simulink model "GFL_mask"  (R2024b)
settings: Solver=ode3  StartTime=0.0  StopTime=20  FixedStep=1e-5  RelTol=1e-3  EnableMultiTasking=on
InitFcn:
  | Ts=5e-6;
values from neighbouring files (symbols this model uses):
  c_f = 0.06    [GFL_compare.m]    (also in dqscan.m; fun00_GFL_pu_2_normial.m = c_f*Cb; fun01_GFL_Small_Signal.m = c_f*Cb)
  fb = 60    [GFL_compare.m]    (also in dqscan.m)
  fpt = fp1    [dqscan.m]
  ki_i = ki_i_pu*Vb_p_ph/Ib_p_ph    [fun00_GFL_pu_2_normial.m]    (also in fun01_GFL_Small_Signal.m)
  ki_p = ki_p_pu/Sb*Ib_p_ph    [fun00_GFL_pu_2_normial.m]    (also in fun01_GFL_Small_Signal.m)
  ki_pll = 377.7    [GFL_compare.m]    (also in dqscan.m; fun00_GFL_pu_2_normial.m = ki_pll/Vb_p_ph; fun01_GFL_Small_Signal.m = ki_pll/Vb_p_ph)
  ki_q = ki_q_pu/Sb*Ib_p_ph    [fun00_GFL_pu_2_normial.m]    (also in fun01_GFL_Small_Signal.m)
  kp_i = kp_i_pu*Vb_p_ph/Ib_p_ph    [fun00_GFL_pu_2_normial.m]    (also in fun01_GFL_Small_Signal.m)
  kp_p = kp_p_pu/Sb*Ib_p_ph    [fun00_GFL_pu_2_normial.m]    (also in fun01_GFL_Small_Signal.m)
  kp_pll = 27.5    [GFL_compare.m]    (also in dqscan.m; fun00_GFL_pu_2_normial.m = kp_pll/Vb_p_ph; fun01_GFL_Small_Signal.m = kp_pll/Vb_p_ph)
  kp_q = kp_q_pu/Sb*Ib_p_ph    [fun00_GFL_pu_2_normial.m]    (also in fun01_GFL_Small_Signal.m)
  l_f = 0.05    [GFL_compare.m]    (also in dqscan.m; fun00_GFL_pu_2_normial.m = l_f*Lb; fun01_GFL_Small_Signal.m = l_f*Lb)
  pset = p_set_pu*Sb    [fun00_GFL_pu_2_normial.m]    (also in fun01_GFL_Small_Signal.m)
  qset = q_set_pu*Sb    [fun00_GFL_pu_2_normial.m]    (also in fun01_GFL_Small_Signal.m)
  r_f = 0.01    [GFL_compare.m]    (also in dqscan.m; fun00_GFL_pu_2_normial.m = r_f*Zb; fun01_GFL_Small_Signal.m = r_f*Zb)
  Sb = 50*10^3    (= 50000)    [GFL_compare.m]    (also in dqscan.m)
  Upd = 0    [dqscan.m]
  Upq = 10    [dqscan.m]
  Vb = 690    [GFL_compare.m]    (also in dqscan.m)
  Vdc = 3*Vb_p_ph    [fun00_GFL_pu_2_normial.m]
  w_b = fb*2*pi    (= 376.991118431)    [GFL_compare.m]    (also in dqscan.m; fun00_GFL_pu_2_normial.m = fb*2*pi; fun01_GFL_Small_Signal.m = fb*2*pi)
undefined symbols (not defined in the file or in its folder): DiscIntNeverNeededParam
libraries: spsabctodq0Lib x10, spsThreePhaseVIMeasurementLib x6, slpidlib x5, spsControlledVoltageSourceLib x3, spsThreePhaseSeriesRLCBranchLib x3, spsGroundLib x2, spsdq0toabcLib x2, spsPowerPositiveSequenceLib x1, spsUniversalBridgeLib x1, spsDCVoltageSourceLib x1, spsPLL3phLib x1, spsThreePhaseProgrammableVoltageSourceLib x1
settings Model: SimulationMode=accelerator  Creator=GeZicheng  LastModifiedBy=PEESE_hmqrtt2
settings DataIOCC: SaveFinalState=on  SaveFormat=StructureWithTime  SaveOutput=off  SignalLogging=off  SaveTime=off  ReturnWorkspaceOutputs=off

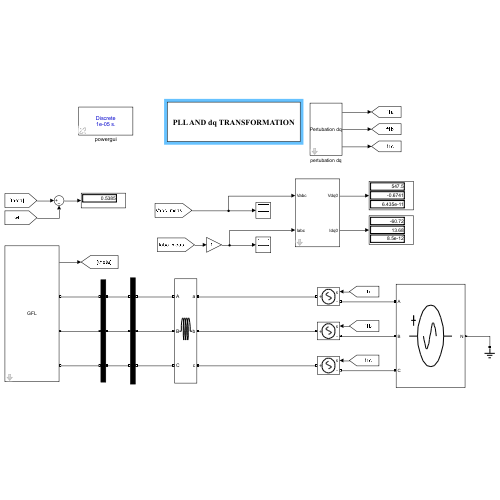
[thumbnail: Simulink's stored preview of the top-level diagram]
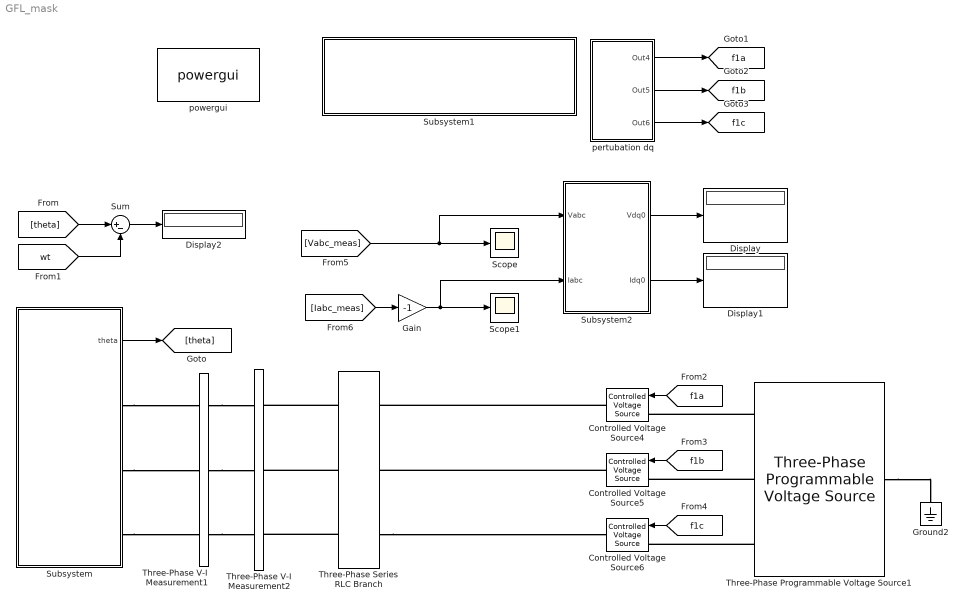
== system GFL_mask ==
  Controlled Voltage Source4 : spsControlledVoltageSourceLib/Controlled Voltage Source  Initialize=on  Source_Type=AC  Amplitude=0  Phase=0  Frequency=0  Measurements=None
  Controlled Voltage Source5 : spsControlledVoltageSourceLib/Controlled Voltage Source  Initialize=on  Source_Type=AC  Amplitude=0  Phase=0  Frequency=0  Measurements=None
  Controlled Voltage Source6 : spsControlledVoltageSourceLib/Controlled Voltage Source  Initialize=on  Source_Type=AC  Amplitude=0  Phase=0  Frequency=0  Measurements=None
  Display : Display
  Display1 : Display
  Display2 : Display
  Gain : Gain  Gain=-1
  Ground2 : spsGroundLib/Ground  LConnTagsString=a
  Scope : Scope
  Scope1 : Scope
  Subsystem : Subsystem  mask{Pnom=Sb, Vnom=Vb, Fnom=fb, Vdc_nom=Vdc, RLC_Filter=[r_f l_f c_f], Pref=pset, Qref=qset, PLL_p=kp_pll, PLL_i=ki_pll, Voltage_P=kp_q, Voltage_I=ki_q, Current_P=kp_i, Current_I=ki_i, Power_P=kp_p, Power_I=ki_p, kf=0.5}
      mask prompts: Pnom "Rated Power(VA)"; Vnom "Rated L-L RMS Voltage(V)"; Fnom "Rated Frequency(Hz)"; Vdc_nom "DC capacitor voltage(V)"; RLC_Filter "Grid-side coupling impedance(p.u.)"; Pref "Power Setting"; Qref "Voltage Setting"; PLL_p "PL Proportional Gain"; PLL_i "PLL Integral Gain"; Voltage_P "Voltage Proportional Gain"; Voltage_I "Voltage Integral Gain"; Current_P "Current Proportional Gain"; Current_I "Current Integral Gain"; Power_P "Power Proportional Gain"; Power_I "Power Integral Gain"; kf "Feedforward Gain"
      mask init:
      | R_f=RLC_Filter(1);
      | L_f=RLC_Filter(2);
      | C_f=RLC_Filter(3);
      mask Display: disp('GFL')
  Subsystem1 : Subsystem
      mask Display: disp('PLL AND dq TRANSFORMATION')
  Subsystem2 : Subsystem
      mask DialogControl ParameterGroupVar Prompt: 参数
  Sum : Sum  Inputs=|+-
  Three-Phase Programmable Voltage Source1 : spsThreePhaseProgrammableVoltageSourceLib/Three-Phase Programmable Voltage Source  PositiveSequence=[Vb 90 fb]  VariationEntity=None  VariationType=Table of time-amplitude pairs  VariationTypeAlt=Step  VariationStep=0.5  VariationRate=10  VariationMagnitude=0.3  VariationFrequency=2  VariationTiming=[1 2]  VariationPhaseA=off  Amplitudes=[1 0.8 1.2 1.0]  TimeValues=[0 0.1 0.15 0.2]  HarmonicGeneration=off  HarmonicA=[3 0.2 -25 0]  HarmonicB=[2 0.15 35 2]  Timing="[0.05  3]"  BusType=swing  Pref=0  Qref=0  Qmin=-inf  Qmax=inf
  Three-Phase Series RLC Branch : spsThreePhaseSeriesRLCBranchLib/Three-Phase Series RLC Branch  LConnTagsString=A|B|C  RConnTagsString=A|B|C  BranchType=L  Resistance=r_f  Inductance=10*l_f  Capacitance=1e-6  Measurements=None
  Three-Phase V-I Measurement1 : spsThreePhaseVIMeasurementLib/Three-Phase V-I Measurement  VoltageMeasurement=phase-to-ground  SetLabelV=on  LabelV=Vabc_o  Vpu=off  VpuLL=off  CurrentMeasurement=yes  SetLabelI=on  LabelI=Iabc_o  Ipu=off  Pbase=100e6  Vbase=500e3  OutputType=Complex  PhasorSimulation=off  PSBequivalent=0
  Three-Phase V-I Measurement2 : spsThreePhaseVIMeasurementLib/Three-Phase V-I Measurement  VoltageMeasurement=phase-to-ground  SetLabelV=on  LabelV=Vabc_meas  Vpu=off  VpuLL=off  CurrentMeasurement=yes  SetLabelI=on  LabelI=Iabc_meas  Ipu=off  Pbase=100e6  Vbase=500e3  OutputType=Complex  PhasorSimulation=off  PSBequivalent=0
  pertubation dq : Subsystem
      mask DialogControl ParameterGroupVar Prompt: 参数
      mask Display: disp('Pertubation dq')
  powergui : spspowerguiLib/powergui  SimulationMode=Discrete  SampleTime=1e-5  frequency=50  Iterations=50  frequencyindice=0  Pbase=100e6  ErrMax=1e-4  UnitsV=kV  UnitsW=MW  buscounter=0  FunctionMessages=off  echomessages=off  EnableUseOfTLC=off  CurrentSourceSwitches=on  DisableSnubberDevices=off  DisableRonSwitches=off  DisableVfSwitches=off  DisplayEquations=off  AutomaticDiscreteSolvers=off  SolverType=Tustin/Backward Euler (TBE)  Interpol=off  ExternalGateDelay=off  methode=off  Ts=0  x0status=blocks  SPID=off  SwTol=0  HookPort=off  NonlinearTolerance=1e-4  nMaxIteration=100  ContinueOnMaxIteration=off  RestoreLinks=warning  ResistiveCurrentMeasurement=off  Frange=[0:2:500]  Ylog=off  Xlog=on  ShowGrid=off  save=off  variable=ZData  structure=0  ZoomFFT=on  StartTime=0.0  cycles=1  DisplayStyle=1  fundamental=60  FreqAxis=off  MaxFrequency=1000  frequencyindicesteady=1  RmsSteady=1  display=off
  tag scope: f1a=global, f1b=global, f1c=global
  wires:
  [Vabc_meas] -> Subsystem2/1(Vabc), Scope/1
  [f1c] -> Controlled Voltage Source6/1
  [f1b] -> Controlled Voltage Source5/1
  [f1a] -> Controlled Voltage Source4/1
  pertubation dq/3(Out6) -> [f1c]
  pertubation dq/1(Out4) -> [f1a]
  pertubation dq/2(Out5) -> [f1b]
  Subsystem2/1(Vdq0) -> Display/1
  Subsystem2/2(Idq0) -> Display1/1
  Gain/1 -> Subsystem2/2(Iabc), Scope1/1
  [theta] -> Sum/1
  [wt] -> Sum/2
  Sum/1 -> Display2/1
  Subsystem/1(theta) -> [theta]
  [Iabc_meas] -> Gain/1
  connections:
  Three-Phase V-I Measurement1/RConn1 -- Three-Phase V-I Measurement2/LConn1
  Three-Phase V-I Measurement1/RConn2 -- Three-Phase V-I Measurement2/LConn2
  Three-Phase V-I Measurement1/RConn3 -- Three-Phase V-I Measurement2/LConn3
  Three-Phase Programmable Voltage Source1/RConn1 -- Controlled Voltage Source4/LConn1
  Three-Phase Programmable Voltage Source1/RConn2 -- Controlled Voltage Source5/LConn1
  Three-Phase Programmable Voltage Source1/RConn3 -- Controlled Voltage Source6/LConn1
  Three-Phase Programmable Voltage Source1/LConn1 -- Ground2/LConn1
  Subsystem/RConn1 -- Three-Phase V-I Measurement1/LConn1
  Subsystem/RConn2 -- Three-Phase V-I Measurement1/LConn2
  Subsystem/RConn3 -- Three-Phase V-I Measurement1/LConn3
  Three-Phase Series RLC Branch/RConn3 -- Controlled Voltage Source6/RConn1
  Controlled Voltage Source5/RConn1 -- Three-Phase Series RLC Branch/RConn2
  Controlled Voltage Source4/RConn1 -- Three-Phase Series RLC Branch/RConn1
  Three-Phase Series RLC Branch/LConn1 -- Three-Phase V-I Measurement2/RConn1
  Three-Phase Series RLC Branch/LConn2 -- Three-Phase V-I Measurement2/RConn2
  Three-Phase Series RLC Branch/LConn3 -- Three-Phase V-I Measurement2/RConn3

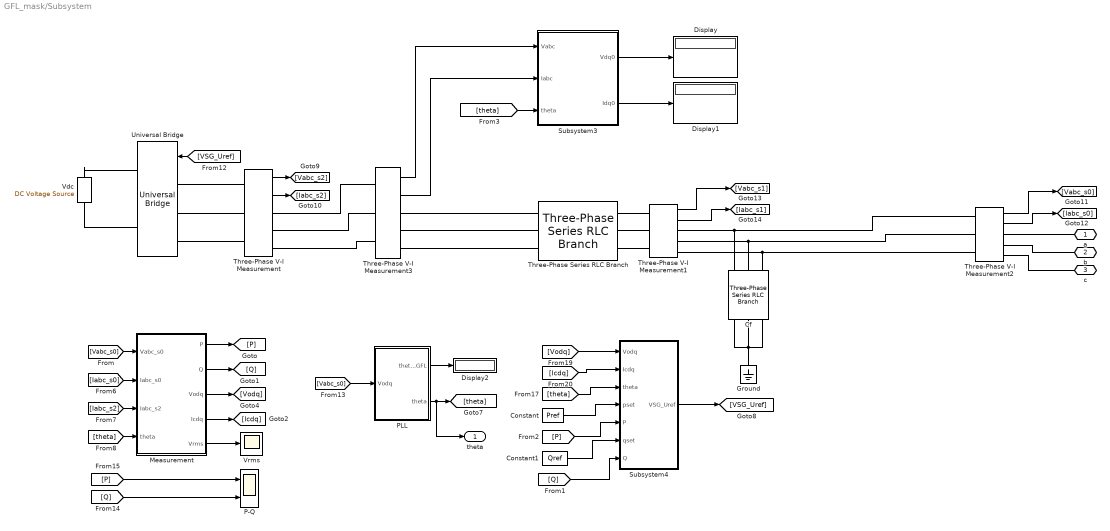
== system GFL_mask/Subsystem ==
  Cf : spsThreePhaseSeriesRLCBranchLib/Three-Phase Series RLC Branch  LConnTagsString=A|B|C  RConnTagsString=A|B|C  BranchType=C  Resistance=0.1  Inductance=1e-3  Capacitance=RLC_Filter(3)  Measurements=None
  Constant : Constant  Value=Pref
  Constant1 : Constant  Value=Qref
  Display : Display
  Display1 : Display
  Display2 : Display
  Ground : spsGroundLib/Ground  LConnTagsString=a
  Measurement : Subsystem
      mask DialogControl ParameterGroupVar Prompt: 参数
  P-Q : Scope  NumInputPorts=2
  PLL : Subsystem
      mask DialogControl ParameterGroupVar Prompt: 参数
  Subsystem3 : Subsystem
      mask DialogControl ParameterGroupVar Prompt: 参数
  Subsystem4 : Subsystem  mask{Voltage_P=Voltage_P, Voltage_I=Voltage_I, Current_P=Current_P, Current_I=Current_I, Power_P=Power_P, Power_I=Power_I, kf=kf}
      mask prompts: Voltage_P "Voltage Proportional Coefficient"; Voltage_I "Voltage Integral Coefficient"; Current_P "Current Proportional Coefficient"; Current_I "Current Integral Coefficient"; Power_P "Power Proportional Coefficient"; Power_I "Power Integral Coefficient"; kf "Feedforward Coeffcient"
      mask DialogControl ParameterGroupVar Prompt: Controller Parameter
  Three-Phase Series RLC Branch : spsThreePhaseSeriesRLCBranchLib/Three-Phase Series RLC Branch  LConnTagsString=A|B|C  RConnTagsString=A|B|C  BranchType=RL  Resistance=RLC_Filter(1)  Inductance=RLC_Filter(2)  Capacitance=1e-6  Measurements=None
  Three-Phase V-I Measurement : spsThreePhaseVIMeasurementLib/Three-Phase V-I Measurement  VoltageMeasurement=phase-to-ground  SetLabelV=off  LabelV=Vabc_s2  Vpu=off  VpuLL=off  CurrentMeasurement=yes  SetLabelI=off  LabelI=Iabc_s2  Ipu=off  Pbase=Pnom  Vbase=Vnom  OutputType=Complex  PhasorSimulation=off  PSBequivalent=0
  Three-Phase V-I Measurement1 : spsThreePhaseVIMeasurementLib/Three-Phase V-I Measurement  VoltageMeasurement=phase-to-ground  SetLabelV=off  LabelV=Vabc_s1  Vpu=off  VpuLL=off  CurrentMeasurement=yes  SetLabelI=off  LabelI=Iabc_s1  Ipu=off  Pbase=Pnom  Vbase=Vnom  OutputType=Complex  PhasorSimulation=off  PSBequivalent=0
  Three-Phase V-I Measurement2 : spsThreePhaseVIMeasurementLib/Three-Phase V-I Measurement  VoltageMeasurement=phase-to-ground  SetLabelV=off  LabelV=Vabc_s0  Vpu=off  VpuLL=off  CurrentMeasurement=yes  SetLabelI=off  LabelI=Iabc_s0  Ipu=off  Pbase=Pnom  Vbase=Vnom  OutputType=Complex  PhasorSimulation=off  PSBequivalent=0
  Three-Phase V-I Measurement3 : spsThreePhaseVIMeasurementLib/Three-Phase V-I Measurement  VoltageMeasurement=phase-to-ground  SetLabelV=off  LabelV=Vabc_s2  Vpu=off  VpuLL=off  CurrentMeasurement=yes  SetLabelI=off  LabelI=Iabc_s2  Ipu=off  Pbase=Pnom  Vbase=Vnom  OutputType=Complex  PhasorSimulation=off  PSBequivalent=0
  Universal Bridge : spsUniversalBridgeLib/Universal Bridge  Arms=3  SnubberResistance=1e5  SnubberCapacitance=inf  Device=Average-model based VSC  Ron=1e-3  Lon=0  ForwardVoltages="[  0  0  ]"  ForwardVoltage=0  GTOparameters=[ 10e-6 , 20e-6 ]  IGBTparameters=[ 1e-6 , 2e-6 ]  Measurements=None  Measurements_2=None  converterType=Rectifier
  Vdc : spsDCVoltageSourceLib/DC Voltage Source  Amplitude=Vdc_nom  Measurements=None
  Vrms : Scope
  a : PMIOPort  Side=Right
  b : PMIOPort  Port=2  Side=Right
  c : PMIOPort  Port=3  Side=Right
  theta : Outport
  wires:
  Measurement/5(Vrms) -> Vrms/1
  Measurement/1(P) -> [P]
  Measurement/2(Q) -> [Q]
  Measurement/3(Vodq) -> [Vodq]
  Measurement/4(Icdq) -> [Icdq]
  [Vabc_s0] -> Measurement/1(Vabc_s0)
  [theta] -> Measurement/4(theta)
  [Iabc_s2] -> Measurement/3(Iabc_s2)
  [Iabc_s0] -> Measurement/2(Iabc_s0)
  [VSG_Uref] -> Universal Bridge/1
  [Vabc_s0] -> PLL/1(Vodq)
  PLL/1(theta_GFL) -> Display2/1
  [P] -> P-Q/1
  [Q] -> P-Q/2
  Three-Phase V-I Measurement3/1 -> Subsystem3/1(Vabc)
  Three-Phase V-I Measurement3/2 -> Subsystem3/2(Iabc)
  Subsystem3/1(Vdq0) -> Display/1
  Subsystem3/2(Idq0) -> Display1/1
  PLL/2(theta) -> theta/1, [theta]
  [Icdq] -> Subsystem4/2(Icdq)
  [Vodq] -> Subsystem4/1(Vodq)
  [theta] -> Subsystem4/3(theta)
  Subsystem4/1(VSG_Uref) -> [VSG_Uref]
  Three-Phase V-I Measurement/1 -> [Vabc_s2]
  Three-Phase V-I Measurement/2 -> [Iabc_s2]
  Three-Phase V-I Measurement2/1 -> [Vabc_s0]
  Three-Phase V-I Measurement2/2 -> [Iabc_s0]
  Three-Phase V-I Measurement1/2 -> [Iabc_s1]
  Three-Phase V-I Measurement1/1 -> [Vabc_s1]
  [P] -> Subsystem4/5(P)
  Constant/1 -> Subsystem4/4(pset)
  Constant1/1 -> Subsystem4/6(qset)
  [theta] -> Subsystem3/3(theta)
  [Q] -> Subsystem4/7(Q)
  connections:
  Cf/LConn2 -- Three-Phase V-I Measurement2/LConn2 -- Three-Phase V-I Measurement1/RConn2
  Cf/LConn1 -- Three-Phase V-I Measurement2/LConn1 -- Three-Phase V-I Measurement1/RConn1
  Cf/LConn3 -- Three-Phase V-I Measurement2/LConn3 -- Three-Phase V-I Measurement1/RConn3
  Three-Phase V-I Measurement1/LConn2 -- Three-Phase Series RLC Branch/RConn2
  Three-Phase V-I Measurement1/LConn1 -- Three-Phase Series RLC Branch/RConn1
  Universal Bridge/RConn2 -- Vdc/LConn1
  Vdc/RConn1 -- Universal Bridge/RConn1
  Three-Phase V-I Measurement/LConn3 -- Universal Bridge/LConn3
  Three-Phase V-I Measurement/LConn2 -- Universal Bridge/LConn2
  Three-Phase V-I Measurement/LConn1 -- Universal Bridge/LConn1
  Three-Phase V-I Measurement1/LConn3 -- Three-Phase Series RLC Branch/RConn3
  Three-Phase V-I Measurement2/RConn1 -- a/RConn1
  Three-Phase V-I Measurement2/RConn2 -- b/RConn1
  Three-Phase V-I Measurement2/RConn3 -- c/RConn1
  Three-Phase V-I Measurement3/RConn1 -- Three-Phase Series RLC Branch/LConn1
  Three-Phase Series RLC Branch/LConn2 -- Three-Phase V-I Measurement3/RConn2
  Three-Phase Series RLC Branch/LConn3 -- Three-Phase V-I Measurement3/RConn3
  Three-Phase V-I Measurement3/LConn1 -- Three-Phase V-I Measurement/RConn1
  Three-Phase V-I Measurement3/LConn2 -- Three-Phase V-I Measurement/RConn2
  Three-Phase V-I Measurement3/LConn3 -- Three-Phase V-I Measurement/RConn3
  Ground/LConn1 -- Cf/RConn2 -- Cf/RConn1 -- Cf/RConn3

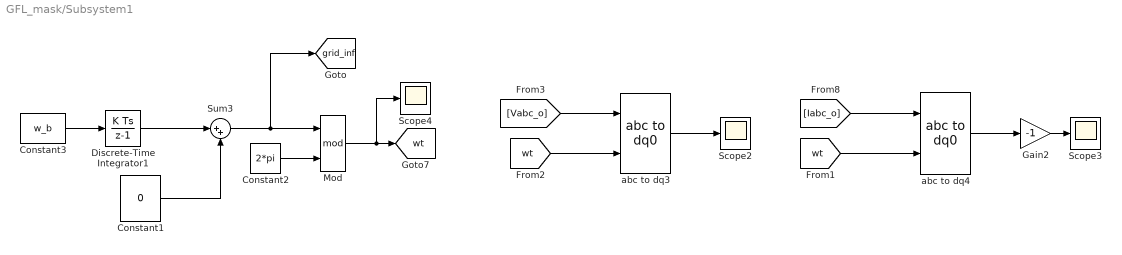
== system GFL_mask/Subsystem1 ==
  Constant1 : Constant  Value=0
  Constant2 : Constant  Value=2*pi
  Constant3 : Constant  Value=w_b
  Discrete-Time Integrator1 : DiscreteIntegrator  SampleTime=-1  ICPrevOutput=DiscIntNeverNeededParam  ICPrevScaledInput=DiscIntNeverNeededParam
  Gain2 : Gain  Gain=-1
  Mod : Math  Operator=mod
  Scope2 : Scope
  Scope3 : Scope
  Scope4 : Scope
  Sum3 : Sum  Inputs=|++
  abc to dq3 : spsabctodq0Lib/abc to dq0  Alignment=Aligned with phase A axis
  abc to dq4 : spsabctodq0Lib/abc to dq0  Alignment=Aligned with phase A axis
  tag scope: grid_inf=global, wt=global
  wires:
  abc to dq4/1 -> Gain2/1
  [wt] -> abc to dq4/2
  abc to dq3/1 -> Scope2/1
  [Iabc_o] -> abc to dq4/1
  [Vabc_o] -> abc to dq3/1
  [wt] -> abc to dq3/2
  Gain2/1 -> Scope3/1
  Sum3/1 -> [grid_inf], Mod/1
  Constant2/1 -> Mod/2
  Constant3/1 -> Discrete-Time Integrator1/1
  Mod/1 -> Scope4/1, [wt]
  Constant1/1 -> Sum3/2
  Discrete-Time Integrator1/1 -> Sum3/1

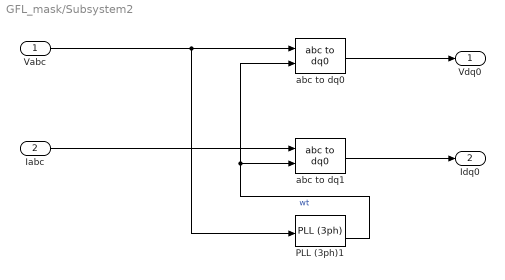
== system GFL_mask/Subsystem2 ==
  Vabc : Inport
  Iabc : Inport  Port=2
  PLL (3ph)1 : spsPLL3phLib/PLL (3ph)  Fmin=fb-5  Par_Init=[0, fb]  ParK=[60, 1400]  TcD=0.04  MaxRateChangeFreq=12  FilterCutOffFreq=25  Ts=0  AGC=on
  abc to dq0 : spsabctodq0Lib/abc to dq0  Alignment=90 degrees behind phase A axis
  abc to dq1 : spsabctodq0Lib/abc to dq0  Alignment=90 degrees behind phase A axis
  Vdq0 : Outport
  Idq0 : Outport  Port=2
  wires:
  abc to dq1/1 -> Idq0/1
  PLL (3ph)1/2 -> abc to dq0/2, abc to dq1/2  "wt"
  abc to dq0/1 -> Vdq0/1
  Iabc/1 -> abc to dq1/1
  Vabc/1 -> PLL (3ph)1/1, abc to dq0/1

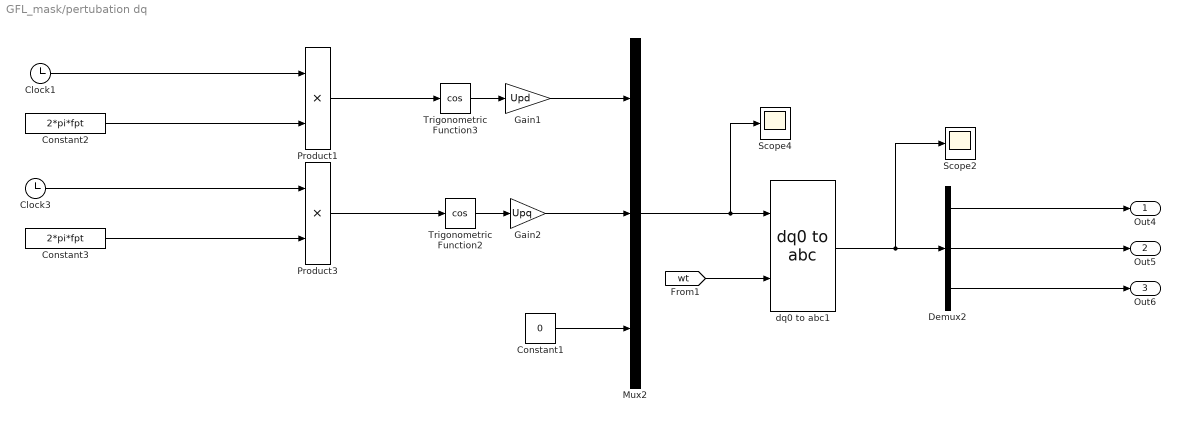
== system GFL_mask/pertubation dq ==
  Clock1 : Clock
  Clock3 : Clock
  Constant1 : Constant  Value=0
  Constant2 : Constant  Value=2*pi*fpt
  Constant3 : Constant  Value=2*pi*fpt
  Demux2 : Demux  Outputs=3
      settings: DisplayOption=none
  Gain1 : Gain  Gain=Upd
  Gain2 : Gain  Gain=Upq
  Mux2 : Mux  Inputs=3
  Product1 : Product
  Product3 : Product
  Scope2 : Scope
  Scope4 : Scope
  Trigonometric Function2 : Trigonometry  Operator=cos
  Trigonometric Function3 : Trigonometry  Operator=cos
  dq0 to abc1 : spsdq0toabcLib/dq0 to abc  Alignment=Aligned with phase A axis
  Out4 : Outport  VectorParamsAs1DForOutWhenUnconnected=off
  Out5 : Outport  Port=2  VectorParamsAs1DForOutWhenUnconnected=off
  Out6 : Outport  Port=3  VectorParamsAs1DForOutWhenUnconnected=off
  wires:
  Demux2/2 -> Out5/1
  dq0 to abc1/1 -> Scope2/1, Demux2/1
  [wt] -> dq0 to abc1/2
  Constant2/1 -> Product1/2
  Demux2/3 -> Out6/1
  Mux2/1 -> Scope4/1, dq0 to abc1/1
  Trigonometric Function3/1 -> Gain1/1
  Constant1/1 -> Mux2/3
  Demux2/1 -> Out4/1
  Gain2/1 -> Mux2/2
  Trigonometric Function2/1 -> Gain2/1
  Gain1/1 -> Mux2/1
  Clock1/1 -> Product1/1
  Product1/1 -> Trigonometric Function3/1
  Clock3/1 -> Product3/1
  Constant3/1 -> Product3/2
  Product3/1 -> Trigonometric Function2/1

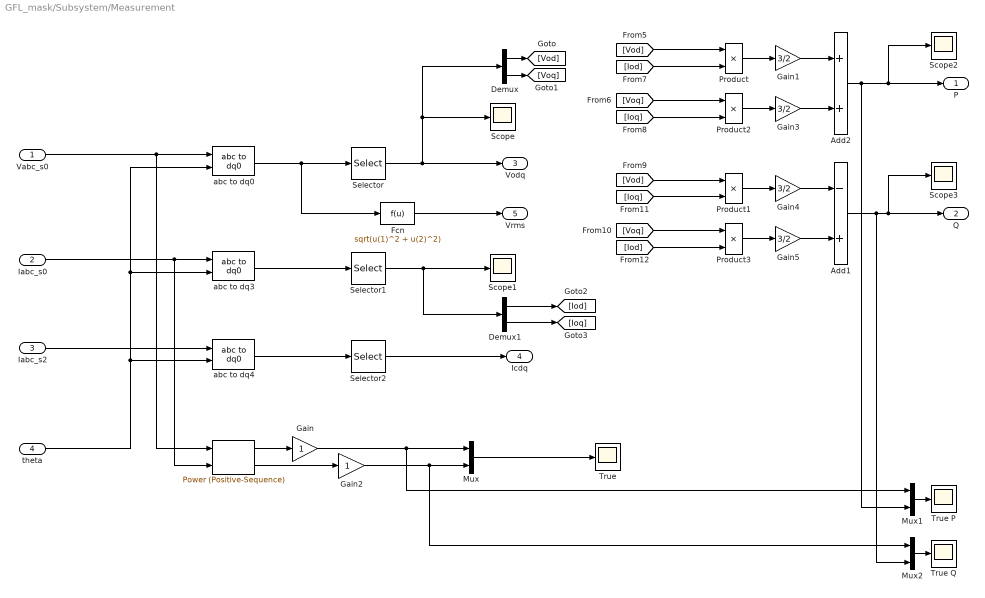
== system GFL_mask/Subsystem/Measurement ==
  Vabc_s0 : Inport
  Iabc_s0 : Inport  Port=2
  Iabc_s2 : Inport  Port=3
  theta : Inport  Port=4
  " " : spsPowerPositiveSequenceLib/Power (Positive-Sequence)  Freq=fb  Vinit=[0, 0]  Iinit=[0, 0]  Ts=0
  Add1 : Sum  Inputs=-+
  Add2 : Sum
  Demux : Demux  Outputs=2
  Demux1 : Demux  Outputs=2
  Fcn : Fcn  Expr=sqrt(u(1)^2 + u(2)^2)
  Gain : Gain
  Gain{1,3..5} (4 alike) : Gain  Gain=3/2
  Gain2 : Gain
  Mux : Mux  Inputs=2
  Mux1 : Mux  Inputs=2
  Mux2 : Mux  Inputs=2
  Product{,1..3} (4 alike) : Product
  Scope{,1..3} (4 alike) : Scope
  Selector : Selector  InputPortWidth=3  IndexOptions=Index vector (dialog)  Indices=[1 2]  OutputSizes=2
  Selector1 : Selector  InputPortWidth=3  IndexOptions=Index vector (dialog)  Indices=[1 2]  OutputSizes=2
  Selector2 : Selector  InputPortWidth=3  IndexOptions=Index vector (dialog)  Indices=[1 2]  OutputSizes=2
  True : Scope
  True P : Scope
  True Q : Scope
  abc to dq0 : spsabctodq0Lib/abc to dq0  Alignment=Aligned with phase A axis
  abc to dq3 : spsabctodq0Lib/abc to dq0  Alignment=Aligned with phase A axis
  abc to dq4 : spsabctodq0Lib/abc to dq0  Alignment=Aligned with phase A axis
  P : Outport
  Q : Outport  Port=2
  Vodq : Outport  Port=3
  Icdq : Outport  Port=4
  Vrms : Outport  Port=5
  wires:
  abc to dq0/1 -> Fcn/1, Selector/1
  theta/1 -> abc to dq4/2, abc to dq3/2, abc to dq0/2
  Add2/1 -> Mux1/2, P/1, Scope2/1
  [Voq] -> Product3/1
  Iabc_s0/1 -> " "/2, abc to dq3/1
  Iabc_s2/1 -> abc to dq4/1
  [Iod] -> Product/2
  [Vod] -> Product1/1
  Selector/1 -> Vodq/1, Demux/1, Scope/1
  [Voq] -> Product2/1
  abc to dq4/1 -> Selector2/1
  [Vod] -> Product/1
  Demux/1 -> [Vod]
  Vabc_s0/1 -> " "/1, abc to dq0/1
  Mux2/1 -> True Q/1
  Fcn/1 -> Vrms/1
  Add1/1 -> Mux2/2, Q/1, Scope3/1
  Mux1/1 -> True P/1
  Selector1/1 -> Demux1/1, Scope1/1
  abc to dq3/1 -> Selector1/1
  Product3/1 -> Gain5/1
  [Ioq] -> Product1/2
  [Iod] -> Product3/2
  Product1/1 -> Gain4/1
  Demux1/2 -> [Ioq]
  Demux1/1 -> [Iod]
  Demux/2 -> [Voq]
  Mux/1 -> True/1
  [Ioq] -> Product2/2
  Selector2/1 -> Icdq/1
  Product2/1 -> Gain3/1
  Product/1 -> Gain1/1
  " "/2 -> Gain2/1
  " "/1 -> Gain/1
  Gain/1 -> Mux1/1, Mux/1
  Gain2/1 -> Mux2/1, Mux/2
  Gain1/1 -> Add2/1
  Gain3/1 -> Add2/2
  Gain4/1 -> Add1/1
  Gain5/1 -> Add1/2

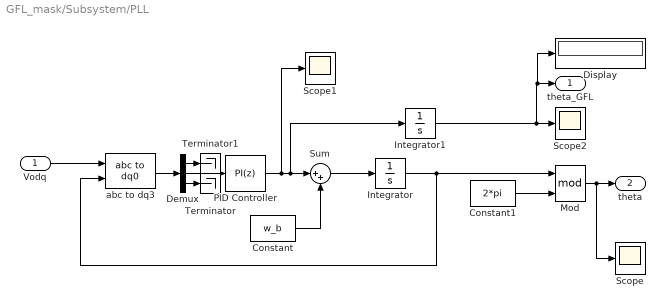
== system GFL_mask/Subsystem/PLL ==
  Vodq : Inport
  Constant : Constant  Value=w_b
  Constant1 : Constant  Value=2*pi
  Demux : Demux  Outputs=3
  Display : Display
  Integrator : Integrator  InitialCondition=w_b
  Integrator1 : Integrator
  Mod : Math  Operator=mod
  PID Controller : slpidlib/PID Controller  Controller=PI  Form=Parallel  TimeDomain=Discrete-time  UseExternalTs=off  SampleTime=-1  IntegratorMethod=Forward Euler  FilterMethod=Forward Euler  ControllerParametersSource=internal  P=PLL_p  I=PLL_i  UseKiTs=off  D=0  UseExternalDerivativeSource=off  N=100  UseFilter=on  TunerSelectOption=Transfer Function Based (PID Tuner App)  ZeroCross=off  InitialConditionSource=internal  InitialConditionForIntegrator=0  InitialConditionForFilter=0  DifferentiatorICPrevScaledInput=0  ExternalReset=none  TrackingMode=off  Kt=1  LimitOutput=off  SatLimitsSource=internal  UpperSaturationLimit=inf  LowerSaturationLimit=-inf  LinearizeAsGain=on  AntiWindupMode=none  Kb=1  LimitIntegrator=off  UpperIntegratorSaturationLimit=inf  LowerIntegratorSaturationLimit=-inf  POutMin=[]  POutMax=[]  IOutMin=[]  IOutMax=[]  DOutMin=[]  DOutMax=[]  NOutMin=[]  NOutMax=[]  SumOutMin=[]  SumOutMax=[]  SaturationOutMin=[]  SaturationOutMax=[]  PParamMin=[]  PParamMax=[]  IParamMin=[]  IParamMax=[]  DParamMin=[]  DParamMax=[]  NParamMin=[]  NParamMax=[]  KbParamMin=[]  KbParamMax=[]  KtParamMin=[]  KtParamMax=[]  KbOutMin=[]  KbOutMax=[]  KtOutMin=[]  KtOutMax=[]  IntegratorOutMin=[]  IntegratorOutMax=[]  FilterOutMin=[]  FilterOutMax=[]  SumI1OutMin=[]  SumI1OutMax=[]  SumI2OutMin=[]  SumI2OutMax=[]  SumI3OutMin=[]  SumI3OutMax=[]  SumI4OutMin=[]  SumI4OutMax=[]  SumDOutMin=[]  SumDOutMax=[]  DifferentiatorOutMin=[]  DifferentiatorOutMax=[]  FilterDiffOutCoefMin=[]  FilterDiffOutCoefMax=[]  ReciprocalOutMin=[]  ReciprocalOutMax=[]  SumDenOutMin=[]  SumDenOutMax=[]  SumNumOutMin=[]  SumNumOutMax=[]  DivideOutMin=[]  DivideOutMax=[]  UdiffTsProdOutMin=[]  UdiffTsProdOutMax=[]  NTsProdOutMin=[]  NTsProdOutMax=[]  UintegralTsProdOutMin=[]  UintegralTsProdOutMax=[]  UngainTsProdOutMin=[]  UngainTsProdOutMax=[]  ClampingZeroOutDataTypeStr=Inherit: Inherit via back propagation  ClampingZeroOutMin=[]  ClampingZeroOutMax=[]  FilterDenConstantOutDataTypeStr=Inherit: Inherit via back propagation  FilterDenConstantOutMin=[]  FilterDenConstantOutMax=[]  PCopyOutDataTypeStr=Inherit: Inherit via back propagation  PCopyOutMin=[]  PCopyOutMax=[]  NCopyOutDataTypeStr=Inherit: Inherit via back propagation  NCopyOutMin=[]  NCopyOutMax=[]  IntegratorContinuousStateAttributes=''  IntegratorStateMustResolveToSignalObject=off  IntegratorRTWStateStorageClass=Auto  FilterContinuousStateAttributes=''  FilterStateMustResolveToSignalObject=off  FilterRTWStateStorageClass=Auto  ParallelPVariant=InternalParameters  IdealPVariant=Disabled  IVariant=InternalParameters  DVariant=Disabled  IntegratorVariant=Discrete  SatVariant=Disabled  AWVariant=Passthrough  PCopyVariant=Disabled  TRVariant=Disabled  FdbkBlocksVariant=Forward  IdealPFdbkVariant=Disabled  SatFdbkVariant=Disabled  DerivativeFilterVariant=Disabled  NVariant=Disabled  NCopyVariant=Disabled_SignalSpec  FilterICVariant=Disabled  IntegratorICVariant=InternalICs  ExternalResetVariant=Disabled  TRSumVariant=Passthrough  SumFdbkVariant=Disabled  SumVariant=Sum_PI  TsampFilterVariant=InternalTs  TsampNgainVariant=Passthrough  TsampIntegralVariant=Disabled_SignalSpec  ExternalSaturationOutDataTypeStr=Inherit: Same as second input  DerivativeSourceVariant=Disabled  PreIntVariant=InternalPreInt
  Scope : Scope
  Scope1 : Scope
  Scope2 : Scope
  Sum : Sum  Inputs=|++
  Terminator : Terminator
  Terminator1 : Terminator
  abc to dq3 : spsabctodq0Lib/abc to dq0  Alignment=Aligned with phase A axis
  theta_GFL : Outport
  theta : Outport  Port=2
  wires:
  Sum/1 -> Integrator/1
  abc to dq3/1 -> Demux/1
  Integrator/1 -> abc to dq3/2, Mod/1
  Constant/1 -> Sum/2
  Integrator1/1 -> Display/1, theta_GFL/1, Scope2/1
  PID Controller/1 -> Scope1/1, Sum/1, Integrator1/1
  Vodq/1 -> abc to dq3/1
  Demux/2 -> PID Controller/1
  Demux/3 -> Terminator/1
  Demux/1 -> Terminator1/1
  Constant1/1 -> Mod/2
  Mod/1 -> Scope/1, theta/1

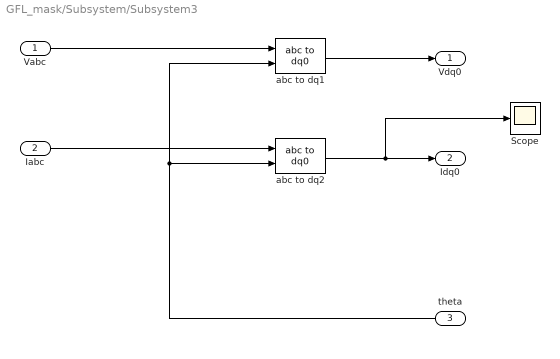
== system GFL_mask/Subsystem/Subsystem3 ==
  Vabc : Inport
  Iabc : Inport  Port=2
  theta : Inport  Port=3
  Scope : Scope
  abc to dq1 : spsabctodq0Lib/abc to dq0  Alignment=Aligned with phase A axis
  abc to dq2 : spsabctodq0Lib/abc to dq0  Alignment=Aligned with phase A axis
  Vdq0 : Outport
  Idq0 : Outport  Port=2
  wires:
  Iabc/1 -> abc to dq2/1
  abc to dq1/1 -> Vdq0/1
  Vabc/1 -> abc to dq1/1
  abc to dq2/1 -> Scope/1, Idq0/1
  theta/1 -> abc to dq2/2, abc to dq1/2

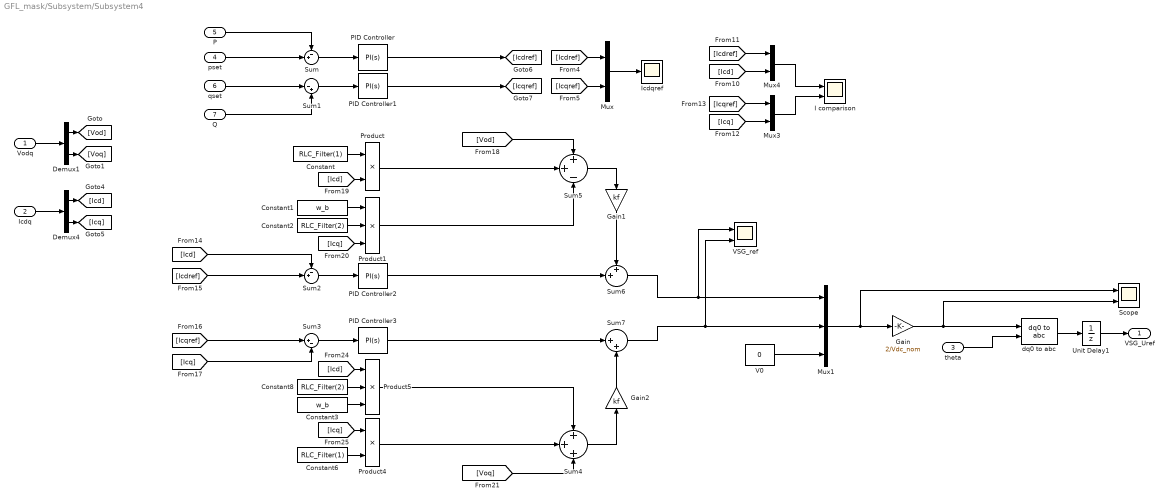
== system GFL_mask/Subsystem/Subsystem4 ==
  Vodq : Inport
  Icdq : Inport  Port=2
  theta : Inport  Port=3
  pset : Inport  Port=4
  P : Inport  Port=5
  qset : Inport  Port=6
  Q : Inport  Port=7
  Constant : Constant  Value=RLC_Filter(1)
  Constant1 : Constant  Value=w_b
  Constant2 : Constant  Value=RLC_Filter(2)
  Constant3 : Constant  Value=w_b
  Constant6 : Constant  Value=RLC_Filter(1)
  Constant8 : Constant  Value=RLC_Filter(2)
  Demux1 : Demux  Outputs=2
  Demux4 : Demux  Outputs=2
  Gain : Gain  Gain=2/Vdc_nom
  Gain1 : Gain  Gain=kf
  Gain2 : Gain  Gain=kf
  I comparison : Scope  NumInputPorts=2
  Icdqref : Scope
  Mux : Mux  Inputs=2
  Mux1 : Mux  Inputs=3
  Mux3 : Mux  Inputs=2
  Mux4 : Mux  Inputs=2
  PID Controller : slpidlib/PID Controller  Controller=PI  Form=Parallel  TimeDomain=Continuous-time  UseExternalTs=off  SampleTime=-1  IntegratorMethod=Forward Euler  FilterMethod=Forward Euler  ControllerParametersSource=internal  P=Power_P  I=Power_I  UseKiTs=off  D=0  UseExternalDerivativeSource=off  N=100  UseFilter=on  TunerSelectOption=Transfer Function Based (PID Tuner App)  InitialConditionSource=internal  InitialConditionForIntegrator=0  InitialConditionForFilter=0  DifferentiatorICPrevScaledInput=0  ExternalReset=none  TrackingMode=off  Kt=1  LimitOutput=off  SatLimitsSource=internal  UpperSaturationLimit=inf  LowerSaturationLimit=-inf  LinearizeAsGain=on  AntiWindupMode=none  Kb=1  LimitIntegrator=off  UpperIntegratorSaturationLimit=inf  LowerIntegratorSaturationLimit=-inf  POutMin=[]  POutMax=[]  IOutMin=[]  IOutMax=[]  DOutMin=[]  DOutMax=[]  NOutMin=[]  NOutMax=[]  SumOutMin=[]  SumOutMax=[]  SaturationOutMin=[]  SaturationOutMax=[]  PParamMin=[]  PParamMax=[]  IParamMin=[]  IParamMax=[]  DParamMin=[]  DParamMax=[]  NParamMin=[]  NParamMax=[]  KbParamMin=[]  KbParamMax=[]  KtParamMin=[]  KtParamMax=[]  KbOutMin=[]  KbOutMax=[]  KtOutMin=[]  KtOutMax=[]  IntegratorOutMin=[]  IntegratorOutMax=[]  FilterOutMin=[]  FilterOutMax=[]  SumI1OutMin=[]  SumI1OutMax=[]  SumI2OutMin=[]  SumI2OutMax=[]  SumI3OutMin=[]  SumI3OutMax=[]  SumI4OutMin=[]  SumI4OutMax=[]  SumDOutMin=[]  SumDOutMax=[]  DifferentiatorOutMin=[]  DifferentiatorOutMax=[]  FilterDiffOutCoefMin=[]  FilterDiffOutCoefMax=[]  ReciprocalOutMin=[]  ReciprocalOutMax=[]  SumDenOutMin=[]  SumDenOutMax=[]  SumNumOutMin=[]  SumNumOutMax=[]  DivideOutMin=[]  DivideOutMax=[]  UdiffTsProdOutMin=[]  UdiffTsProdOutMax=[]  NTsProdOutMin=[]  NTsProdOutMax=[]  UintegralTsProdOutMin=[]  UintegralTsProdOutMax=[]  UngainTsProdOutMin=[]  UngainTsProdOutMax=[]  ClampingZeroOutDataTypeStr=Inherit: Inherit via back propagation  ClampingZeroOutMin=[]  ClampingZeroOutMax=[]  FilterDenConstantOutDataTypeStr=Inherit: Inherit via back propagation  FilterDenConstantOutMin=[]  FilterDenConstantOutMax=[]  PCopyOutDataTypeStr=Inherit: Inherit via back propagation  PCopyOutMin=[]  PCopyOutMax=[]  NCopyOutDataTypeStr=Inherit: Inherit via back propagation  NCopyOutMin=[]  NCopyOutMax=[]  IntegratorContinuousStateAttributes=''  IntegratorStateMustResolveToSignalObject=off  IntegratorRTWStateStorageClass=Auto  FilterContinuousStateAttributes=''  FilterStateMustResolveToSignalObject=off  FilterRTWStateStorageClass=Auto  ParallelPVariant=InternalParameters  IdealPVariant=Disabled  IVariant=InternalParameters  DVariant=Disabled  IntegratorVariant=Continuous  SatVariant=Disabled  AWVariant=Passthrough  PCopyVariant=Disabled  TRVariant=Disabled  FdbkBlocksVariant=Forward  IdealPFdbkVariant=Disabled  SatFdbkVariant=Disabled  DerivativeFilterVariant=Disabled  NVariant=Disabled  NCopyVariant=Disabled_SignalSpec  FilterICVariant=Disabled  IntegratorICVariant=InternalICs  ExternalResetVariant=Disabled  TRSumVariant=Passthrough  SumFdbkVariant=Disabled  SumVariant=Sum_PI  TsampFilterVariant=InternalTs  TsampNgainVariant=Passthrough  TsampIntegralVariant=Disabled_SignalSpec  ExternalSaturationOutDataTypeStr=Inherit: Same as second input  DerivativeSourceVariant=Disabled  PreIntVariant=InternalPreInt
  PID Controller1 : slpidlib/PID Controller  Controller=PI  Form=Parallel  TimeDomain=Continuous-time  UseExternalTs=off  SampleTime=-1  IntegratorMethod=Forward Euler  FilterMethod=Forward Euler  ControllerParametersSource=internal  P=Voltage_P  I=Voltage_I  UseKiTs=off  D=0  UseExternalDerivativeSource=off  N=100  UseFilter=on  TunerSelectOption=Transfer Function Based (PID Tuner App)  InitialConditionSource=internal  InitialConditionForIntegrator=0  InitialConditionForFilter=0  DifferentiatorICPrevScaledInput=0  ExternalReset=none  TrackingMode=off  Kt=1  LimitOutput=off  SatLimitsSource=internal  UpperSaturationLimit=inf  LowerSaturationLimit=-inf  LinearizeAsGain=on  AntiWindupMode=none  Kb=1  LimitIntegrator=off  UpperIntegratorSaturationLimit=inf  LowerIntegratorSaturationLimit=-inf  POutMin=[]  POutMax=[]  IOutMin=[]  IOutMax=[]  DOutMin=[]  DOutMax=[]  NOutMin=[]  NOutMax=[]  SumOutMin=[]  SumOutMax=[]  SaturationOutMin=[]  SaturationOutMax=[]  PParamMin=[]  PParamMax=[]  IParamMin=[]  IParamMax=[]  DParamMin=[]  DParamMax=[]  NParamMin=[]  NParamMax=[]  KbParamMin=[]  KbParamMax=[]  KtParamMin=[]  KtParamMax=[]  KbOutMin=[]  KbOutMax=[]  KtOutMin=[]  KtOutMax=[]  IntegratorOutMin=[]  IntegratorOutMax=[]  FilterOutMin=[]  FilterOutMax=[]  SumI1OutMin=[]  SumI1OutMax=[]  SumI2OutMin=[]  SumI2OutMax=[]  SumI3OutMin=[]  SumI3OutMax=[]  SumI4OutMin=[]  SumI4OutMax=[]  SumDOutMin=[]  SumDOutMax=[]  DifferentiatorOutMin=[]  DifferentiatorOutMax=[]  FilterDiffOutCoefMin=[]  FilterDiffOutCoefMax=[]  ReciprocalOutMin=[]  ReciprocalOutMax=[]  SumDenOutMin=[]  SumDenOutMax=[]  SumNumOutMin=[]  SumNumOutMax=[]  DivideOutMin=[]  DivideOutMax=[]  UdiffTsProdOutMin=[]  UdiffTsProdOutMax=[]  NTsProdOutMin=[]  NTsProdOutMax=[]  UintegralTsProdOutMin=[]  UintegralTsProdOutMax=[]  UngainTsProdOutMin=[]  UngainTsProdOutMax=[]  ClampingZeroOutDataTypeStr=Inherit: Inherit via back propagation  ClampingZeroOutMin=[]  ClampingZeroOutMax=[]  FilterDenConstantOutDataTypeStr=Inherit: Inherit via back propagation  FilterDenConstantOutMin=[]  FilterDenConstantOutMax=[]  PCopyOutDataTypeStr=Inherit: Inherit via back propagation  PCopyOutMin=[]  PCopyOutMax=[]  NCopyOutDataTypeStr=Inherit: Inherit via back propagation  NCopyOutMin=[]  NCopyOutMax=[]  IntegratorContinuousStateAttributes=''  IntegratorStateMustResolveToSignalObject=off  IntegratorRTWStateStorageClass=Auto  FilterContinuousStateAttributes=''  FilterStateMustResolveToSignalObject=off  FilterRTWStateStorageClass=Auto  ParallelPVariant=InternalParameters  IdealPVariant=Disabled  IVariant=InternalParameters  DVariant=Disabled  IntegratorVariant=Continuous  SatVariant=Disabled  AWVariant=Passthrough  PCopyVariant=Disabled  TRVariant=Disabled  FdbkBlocksVariant=Forward  IdealPFdbkVariant=Disabled  SatFdbkVariant=Disabled  DerivativeFilterVariant=Disabled  NVariant=Disabled  NCopyVariant=Disabled_SignalSpec  FilterICVariant=Disabled  IntegratorICVariant=InternalICs  ExternalResetVariant=Disabled  TRSumVariant=Passthrough  SumFdbkVariant=Disabled  SumVariant=Sum_PI  TsampFilterVariant=InternalTs  TsampNgainVariant=Passthrough  TsampIntegralVariant=Disabled_SignalSpec  ExternalSaturationOutDataTypeStr=Inherit: Same as second input  DerivativeSourceVariant=Disabled  PreIntVariant=InternalPreInt
  PID Controller2 : slpidlib/PID Controller  Controller=PI  Form=Parallel  TimeDomain=Continuous-time  UseExternalTs=off  SampleTime=-1  IntegratorMethod=Forward Euler  FilterMethod=Forward Euler  ControllerParametersSource=internal  P=Current_P  I=Current_I  UseKiTs=off  D=0  UseExternalDerivativeSource=off  N=100  UseFilter=on  TunerSelectOption=Transfer Function Based (PID Tuner App)  InitialConditionSource=internal  InitialConditionForIntegrator=0  InitialConditionForFilter=0  DifferentiatorICPrevScaledInput=0  ExternalReset=none  TrackingMode=off  Kt=1  LimitOutput=off  SatLimitsSource=internal  UpperSaturationLimit=inf  LowerSaturationLimit=-inf  LinearizeAsGain=on  AntiWindupMode=none  Kb=1  LimitIntegrator=off  UpperIntegratorSaturationLimit=inf  LowerIntegratorSaturationLimit=-inf  POutMin=[]  POutMax=[]  IOutMin=[]  IOutMax=[]  DOutMin=[]  DOutMax=[]  NOutMin=[]  NOutMax=[]  SumOutMin=[]  SumOutMax=[]  SaturationOutMin=[]  SaturationOutMax=[]  PParamMin=[]  PParamMax=[]  IParamMin=[]  IParamMax=[]  DParamMin=[]  DParamMax=[]  NParamMin=[]  NParamMax=[]  KbParamMin=[]  KbParamMax=[]  KtParamMin=[]  KtParamMax=[]  KbOutMin=[]  KbOutMax=[]  KtOutMin=[]  KtOutMax=[]  IntegratorOutMin=[]  IntegratorOutMax=[]  FilterOutMin=[]  FilterOutMax=[]  SumI1OutMin=[]  SumI1OutMax=[]  SumI2OutMin=[]  SumI2OutMax=[]  SumI3OutMin=[]  SumI3OutMax=[]  SumI4OutMin=[]  SumI4OutMax=[]  SumDOutMin=[]  SumDOutMax=[]  DifferentiatorOutMin=[]  DifferentiatorOutMax=[]  FilterDiffOutCoefMin=[]  FilterDiffOutCoefMax=[]  ReciprocalOutMin=[]  ReciprocalOutMax=[]  SumDenOutMin=[]  SumDenOutMax=[]  SumNumOutMin=[]  SumNumOutMax=[]  DivideOutMin=[]  DivideOutMax=[]  UdiffTsProdOutMin=[]  UdiffTsProdOutMax=[]  NTsProdOutMin=[]  NTsProdOutMax=[]  UintegralTsProdOutMin=[]  UintegralTsProdOutMax=[]  UngainTsProdOutMin=[]  UngainTsProdOutMax=[]  ClampingZeroOutDataTypeStr=Inherit: Inherit via back propagation  ClampingZeroOutMin=[]  ClampingZeroOutMax=[]  FilterDenConstantOutDataTypeStr=Inherit: Inherit via back propagation  FilterDenConstantOutMin=[]  FilterDenConstantOutMax=[]  PCopyOutDataTypeStr=Inherit: Inherit via back propagation  PCopyOutMin=[]  PCopyOutMax=[]  NCopyOutDataTypeStr=Inherit: Inherit via back propagation  NCopyOutMin=[]  NCopyOutMax=[]  IntegratorContinuousStateAttributes=''  IntegratorStateMustResolveToSignalObject=off  IntegratorRTWStateStorageClass=Auto  FilterContinuousStateAttributes=''  FilterStateMustResolveToSignalObject=off  FilterRTWStateStorageClass=Auto  ParallelPVariant=InternalParameters  IdealPVariant=Disabled  IVariant=InternalParameters  DVariant=Disabled  IntegratorVariant=Continuous  SatVariant=Disabled  AWVariant=Passthrough  PCopyVariant=Disabled  TRVariant=Disabled  FdbkBlocksVariant=Forward  IdealPFdbkVariant=Disabled  SatFdbkVariant=Disabled  DerivativeFilterVariant=Disabled  NVariant=Disabled  NCopyVariant=Disabled_SignalSpec  FilterICVariant=Disabled  IntegratorICVariant=InternalICs  ExternalResetVariant=Disabled  TRSumVariant=Passthrough  SumFdbkVariant=Disabled  SumVariant=Sum_PI  TsampFilterVariant=InternalTs  TsampNgainVariant=Passthrough  TsampIntegralVariant=Disabled_SignalSpec  ExternalSaturationOutDataTypeStr=Inherit: Same as second input  DerivativeSourceVariant=Disabled  PreIntVariant=InternalPreInt
  PID Controller3 : slpidlib/PID Controller  Controller=PI  Form=Parallel  TimeDomain=Continuous-time  UseExternalTs=off  SampleTime=-1  IntegratorMethod=Forward Euler  FilterMethod=Forward Euler  ControllerParametersSource=internal  P=Current_P  I=Current_I  UseKiTs=off  D=0  UseExternalDerivativeSource=off  N=100  UseFilter=on  TunerSelectOption=Transfer Function Based (PID Tuner App)  InitialConditionSource=internal  InitialConditionForIntegrator=0  InitialConditionForFilter=0  DifferentiatorICPrevScaledInput=0  ExternalReset=none  TrackingMode=off  Kt=1  LimitOutput=off  SatLimitsSource=internal  UpperSaturationLimit=inf  LowerSaturationLimit=-inf  LinearizeAsGain=on  AntiWindupMode=none  Kb=1  LimitIntegrator=off  UpperIntegratorSaturationLimit=inf  LowerIntegratorSaturationLimit=-inf  POutMin=[]  POutMax=[]  IOutMin=[]  IOutMax=[]  DOutMin=[]  DOutMax=[]  NOutMin=[]  NOutMax=[]  SumOutMin=[]  SumOutMax=[]  SaturationOutMin=[]  SaturationOutMax=[]  PParamMin=[]  PParamMax=[]  IParamMin=[]  IParamMax=[]  DParamMin=[]  DParamMax=[]  NParamMin=[]  NParamMax=[]  KbParamMin=[]  KbParamMax=[]  KtParamMin=[]  KtParamMax=[]  KbOutMin=[]  KbOutMax=[]  KtOutMin=[]  KtOutMax=[]  IntegratorOutMin=[]  IntegratorOutMax=[]  FilterOutMin=[]  FilterOutMax=[]  SumI1OutMin=[]  SumI1OutMax=[]  SumI2OutMin=[]  SumI2OutMax=[]  SumI3OutMin=[]  SumI3OutMax=[]  SumI4OutMin=[]  SumI4OutMax=[]  SumDOutMin=[]  SumDOutMax=[]  DifferentiatorOutMin=[]  DifferentiatorOutMax=[]  FilterDiffOutCoefMin=[]  FilterDiffOutCoefMax=[]  ReciprocalOutMin=[]  ReciprocalOutMax=[]  SumDenOutMin=[]  SumDenOutMax=[]  SumNumOutMin=[]  SumNumOutMax=[]  DivideOutMin=[]  DivideOutMax=[]  UdiffTsProdOutMin=[]  UdiffTsProdOutMax=[]  NTsProdOutMin=[]  NTsProdOutMax=[]  UintegralTsProdOutMin=[]  UintegralTsProdOutMax=[]  UngainTsProdOutMin=[]  UngainTsProdOutMax=[]  ClampingZeroOutDataTypeStr=Inherit: Inherit via back propagation  ClampingZeroOutMin=[]  ClampingZeroOutMax=[]  FilterDenConstantOutDataTypeStr=Inherit: Inherit via back propagation  FilterDenConstantOutMin=[]  FilterDenConstantOutMax=[]  PCopyOutDataTypeStr=Inherit: Inherit via back propagation  PCopyOutMin=[]  PCopyOutMax=[]  NCopyOutDataTypeStr=Inherit: Inherit via back propagation  NCopyOutMin=[]  NCopyOutMax=[]  IntegratorContinuousStateAttributes=''  IntegratorStateMustResolveToSignalObject=off  IntegratorRTWStateStorageClass=Auto  FilterContinuousStateAttributes=''  FilterStateMustResolveToSignalObject=off  FilterRTWStateStorageClass=Auto  ParallelPVariant=InternalParameters  IdealPVariant=Disabled  IVariant=InternalParameters  DVariant=Disabled  IntegratorVariant=Continuous  SatVariant=Disabled  AWVariant=Passthrough  PCopyVariant=Disabled  TRVariant=Disabled  FdbkBlocksVariant=Forward  IdealPFdbkVariant=Disabled  SatFdbkVariant=Disabled  DerivativeFilterVariant=Disabled  NVariant=Disabled  NCopyVariant=Disabled_SignalSpec  FilterICVariant=Disabled  IntegratorICVariant=InternalICs  ExternalResetVariant=Disabled  TRSumVariant=Passthrough  SumFdbkVariant=Disabled  SumVariant=Sum_PI  TsampFilterVariant=InternalTs  TsampNgainVariant=Passthrough  TsampIntegralVariant=Disabled_SignalSpec  ExternalSaturationOutDataTypeStr=Inherit: Same as second input  DerivativeSourceVariant=Disabled  PreIntVariant=InternalPreInt
  Product : Product
  Product1 : Product  Inputs=3
  Product4 : Product
  Product5 : Product  Inputs=3
  Scope : Scope  NumInputPorts=2
  Sum : Sum  Inputs=-+|
  Sum1 : Sum  Inputs=|-+
  Sum2 : Sum  Inputs=-+|
  Sum3 : Sum  Inputs=|+-
  Sum4 : Sum  Inputs=+++
  Sum5 : Sum  Inputs=++-
  Sum6 : Sum  Inputs=++|
  Sum7 : Sum  Inputs=|++
  Unit Delay1 : UnitDelay  SampleTime=-1  HasFrameUpgradeWarning=on
  V0 : Constant  Value=0
  VSG_ref : Scope  NumInputPorts=2
  dq0 to abc : spsdq0toabcLib/dq0 to abc  Alignment=Aligned with phase A axis
  VSG_Uref : Outport
  wires:
  Sum/1 -> PID Controller/1
  Sum1/1 -> PID Controller1/1
  PID Controller/1 -> [Icdref]
  PID Controller1/1 -> [Icqref]
  Mux/1 -> Icdqref/1
  Mux4/1 -> I comparison/1
  Mux1/1 -> Scope/1, Gain/1
  Vodq/1 -> Demux1/1
  Demux1/1 -> [Vod]
  Demux1/2 -> [Voq]
  Demux4/1 -> [Icd]
  Icdq/1 -> Demux4/1
  Demux4/2 -> [Icq]
  [Icdref] -> Mux/1
  [Icqref] -> Mux/2
  [Icd] -> Mux4/2
  [Icdref] -> Mux4/1
  [Icqref] -> Mux3/1
  [Icq] -> Mux3/2
  Mux3/1 -> I comparison/2
  [Icd] -> Sum2/1
  Sum2/1 -> PID Controller2/1
  Sum3/1 -> PID Controller3/1
  [Vod] -> Sum5/1
  Constant/1 -> Product/1
  [Icd] -> Product/2
  Product/1 -> Sum5/2
  Constant1/1 -> Product1/1
  Constant2/1 -> Product1/2
  [Icq] -> Product1/3
  Product1/1 -> Sum5/3
  Constant6/1 -> Product4/2
  [Icq] -> Product4/1
  [Icd] -> Product5/1
  Constant8/1 -> Product5/2
  Constant3/1 -> Product5/3
  V0/1 -> Mux1/3
  theta/1 -> dq0 to abc/2
  PID Controller2/1 -> Sum6/2
  Sum5/1 -> Gain1/1
  Product5/1 -> Sum4/1
  Product4/1 -> Sum4/2
  [Voq] -> Sum4/3
  PID Controller3/1 -> Sum7/1
  Sum4/1 -> Gain2/1
  Sum7/1 -> Mux1/2, VSG_ref/2
  Sum6/1 -> Mux1/1, VSG_ref/1
  dq0 to abc/1 -> Unit Delay1/1
  pset/1 -> Sum/2
  P/1 -> Sum/1
  [Icq] -> Sum3/2
  [Icdref] -> Sum2/2
  [Icqref] -> Sum3/1
  Unit Delay1/1 -> VSG_Uref/1
  Gain/1 -> dq0 to abc/1, Scope/2
  Gain1/1 -> Sum6/1
  Gain2/1 -> Sum7/2
  qset/1 -> Sum1/1
  Q/1 -> Sum1/2
